simulink model "W1P4_model"  (R2020a)
settings: Solver=VariableStepAuto  StartTime=0.0  StopTime=10.0  RelTol=1e-3
settings Model: Creator=avn19  LastModifiedBy=avn19

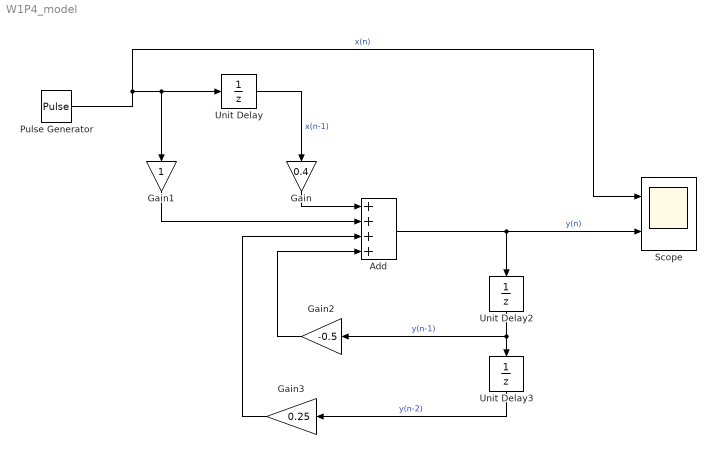
== system W1P4_model ==
  Add : Sum  Inputs=++++
  Gain : Gain  Gain=0.4
  Gain1 : Gain
  Gain2 : Gain  Gain=-0.5
  Gain3 : Gain  Gain=0.25
  Pulse Generator : DiscretePulseGenerator  PulseType=Time based  Period=10  PulseWidth=5
  Scope : Scope  NumInputPorts=2
  Unit Delay : UnitDelay  SampleTime=-1  HasFrameUpgradeWarning=on
  Unit Delay2 : UnitDelay  SampleTime=-1  HasFrameUpgradeWarning=on
  Unit Delay3 : UnitDelay  SampleTime=-1  HasFrameUpgradeWarning=on
  wires:
  Unit Delay2/1 -> Unit Delay3/1, Gain2/1  "y(n-1)"
  Gain3/1 -> Add/3
  Pulse Generator/1 -> Unit Delay/1, Gain1/1, Scope/1  "x(n)"
  Gain2/1 -> Add/4
  Unit Delay3/1 -> Gain3/1  "y(n-2)"
  Gain1/1 -> Add/2
  Unit Delay/1 -> Gain/1  "x(n-1)"
  Gain/1 -> Add/1
  Add/1 -> Unit Delay2/1, Scope/2  "y(n)"
